simulink model "auto_pilot_udp"  (R2022b)
settings: Solver=FixedStepAuto  StartTime=0.0  StopTime=Inf  FixedStep=0.001  RelTol=1e-3  EnableMultiTasking=on
InitFcn:
  | clear mex
model workspace (MAT data in the model file):
  worldsim_instance : object (value not decoded)
values from neighbouring files (symbols this model uses):
  ACC_Adaptive_D = 0    [AutoPilot_parameters.m]    (also in ap_ini_param.mat; ap_initialModel.sldd = 0.0)
  ACC_Adaptive_I = 0    [AutoPilot_parameters.m]    (also in ap_ini_param.mat; ap_initialModel.sldd = 0.0)
  ACC_Adaptive_P = [5 7.5]    [AutoPilot_parameters.m]    (also in ap_ini_param.mat; ap_initialModel.sldd = 5.0 7.5)
  ACC_Classic_I = 5    [AutoPilot_parameters.m]    (also in ap_ini_param.mat; ap_initialModel.sldd = 5.0)
  ACC_Classic_P = 15    [AutoPilot_parameters.m]    (also in ap_ini_param.mat; ap_initialModel.sldd = 15.0)
  ACC_MaxBrake = 50    [AutoPilot_parameters.m]    (also in ap_ini_param.mat; ap_initialModel.sldd = 50.0)
  ACC_MaxThrottle = 130    [AutoPilot_parameters.m]    (also in ap_ini_param.mat = 80; ap_initialModel.sldd = 130.0)
  ACC_Module_Activity_Flag = 1    [AutoPilot_parameters.m]    (also in ap_ini_param.mat; ap_initialModel.sldd = 1.0)
  ACC_Ready_Speed = 30    [AutoPilot_parameters.m]    (also in ap_ini_param.mat; ap_initialModel.sldd = 30.0)
  ACC_SensorMaxDistance = 250    [AutoPilot_parameters.m]    (also in ap_ini_param.mat = 120; ap_initialModel.sldd = 250.0)
  ACC_Speed_Distance_control = 3    [AutoPilot_parameters.m]    (also in ap_ini_param.mat; ap_initialModel.sldd = 3.0)
  ACC_Speed_Distance_Gain = [0.1 0.15 0.2 0.25]    [AutoPilot_parameters.m]    (also in ap_ini_param.mat; ap_initialModel.sldd = 0.1 0.15 0.2 0.25)
  ADAS_Control_Mode = 1    [AutoPilot_parameters.m]    (also in ap_ini_param.mat; ap_initialModel.sldd = 1.0)
  AEB_Alarm_Freq = 5    [AutoPilot_parameters.m]    (also in ap_ini_param.mat; ap_initialModel.sldd = 5.0)
  AEB_Distance_To_Collision_Brake = 5    [AutoPilot_parameters.m]    (also in ap_ini_param.mat; ap_initialModel.sldd = 5.0)
  AEB_Freq_Hz = Sensor_Freq_worldsim/2    (= 25)    [AutoPilot_parameters.m]    (also in ap_ini_param.mat; ap_initialModel.sldd = 25.0)
  AEB_Gain = [1 1]    [AutoPilot_parameters.m]    (also in ap_ini_param.mat; ap_initialModel.sldd = 1.0 1.0)
  AEB_Gain_set = 60    [AutoPilot_parameters.m]    (also in ap_ini_param.mat; ap_initialModel.sldd = 60.0)
  AEB_Gain_set_mult = 0.03    [AutoPilot_parameters.m]    (also in ap_ini_param.mat; ap_initialModel.sldd)
  AEB_Max_Decel = [8 15]    [AutoPilot_parameters.m]    (also in ap_ini_param.mat; ap_initialModel.sldd = 8.0 15.0)
  AEB_Max_Speed = 150    [AutoPilot_parameters.m]    (also in ap_ini_param.mat = 100; ap_initialModel.sldd = 150.0)
  AEB_Min_Distance_at_Stop = 1    [AutoPilot_parameters.m]    (also in ap_ini_param.mat; ap_initialModel.sldd = 1.0)
  AEB_Module_Activity_Flag = 1    [AutoPilot_parameters.m]    (also in ap_ini_param.mat; ap_initialModel.sldd = 1.0)
  AEB_Pedestrian_type = 68    [AutoPilot_parameters.m]    (also in ap_ini_param.mat; ap_initialModel.sldd = 68.0)
  AEB_Steer_Max = 180    [AutoPilot_parameters.m]    (also in ap_ini_param.mat; ap_initialModel.sldd = 180.0)
  AP_Activity_Flag = 1    [AutoPilot_parameters.m]    (also in ap_ini_param.mat; ap_initialModel.sldd = 1.0)
  AP_D = [0.3 0.3]    [AutoPilot_parameters.m]    (also in ap_ini_param.mat; ap_initialModel.sldd = 0.3 0.3)
  AP_Dyn_Rate_Limiter_Gain = 0.1    [AutoPilot_parameters.m]    (also in ap_ini_param.mat; ap_initialModel.sldd)
  AP_Dyn_Rate_Limiter_Power = 10    [AutoPilot_parameters.m]    (also in ap_ini_param.mat; ap_initialModel.sldd = 10.0)
  AP_Error_Max = 3    [AutoPilot_parameters.m]    (also in ap_ini_param.mat; ap_initialModel.sldd = 3.0)
  AP_Freq_Hz = Sensor_Freq_worldsim    (= 50)    [AutoPilot_parameters.m]    (also in ap_ini_param.mat; ap_initialModel.sldd = 50.0)
  AP_I = [0.05 0.05]    [AutoPilot_parameters.m]    (also in ap_ini_param.mat; ap_initialModel.sldd = 0.05 0.05)
  AP_Max_Error_dydt_Disable = 0.5    [AutoPilot_parameters.m]    (also in ap_ini_param.mat; ap_initialModel.sldd)
  AP_On_Request_Time = 0.01    [AutoPilot_parameters.m]    (also in ap_ini_param.mat; ap_initialModel.sldd)
  AP_P = [0.2 0.2]    [AutoPilot_parameters.m]    (also in ap_ini_param.mat; ap_initialModel.sldd = 0.2 0.2)
  AP_Steer_Error_Max = 0.7    [AutoPilot_parameters.m]    (also in ap_ini_param.mat; ap_initialModel.sldd)
  AP_Steer_Rate_Max_radps = 1    [AutoPilot_parameters.m]    (also in ap_ini_param.mat; ap_initialModel.sldd = 1.0)
  AP_Transition_Rate = 0.5    [AutoPilot_parameters.m]    (also in ap_ini_param.mat; ap_initialModel.sldd)
  butter_a = [1 -1.9911142922 0.991153595869]    [ap_ini_param.mat]    (also in ap_initialModel.sldd = 1.0 -1.9911142922016536 0.99115359586893548)
  butter_a_lka_out = 1.0 -1.5610180758007179 0.641351538057563    [ap_initialModel.sldd]
  butter_b = [9.82591682048e-06 1.9651833641e-05 9.82591682048e-06]    [ap_ini_param.mat]    (also in ap_initialModel.sldd = 9.825916820482009E-6 1.9651833640964018E-5 9.825916820482009)
  butter_b_lka_out = 0.020083365564211246 0.040166731128422492 0.020083365564211246    [ap_initialModel.sldd]
  Lane_Width = 3.7    [AutoPilot_parameters.m]    (also in ap_ini_param.mat; ap_initialModel.sldd)
  LDW_Activity_Flag = 1    [ap_ini_param.mat]    (also in ap_initialModel.sldd = 1.0)
  LDW_Freq_Hz = 50    [ap_ini_param.mat]    (also in ap_initialModel.sldd = 50.0)
  LDW_LaneGap_dydt_Warning = 50    [ap_ini_param.mat]    (also in ap_initialModel.sldd = 50.0)
  LDW_LaneGap_Warning = [0.5 0.25]    [ap_ini_param.mat]    (also in ap_initialModel.sldd = 0.5 0.25)
  LDW_Min_Speed = 60    [ap_ini_param.mat]    (also in ap_initialModel.sldd = 60.0)
  LDW_Steer_Vibration_Amplitude = 5    [ap_ini_param.mat]    (also in ap_initialModel.sldd = 5.0)
  LDW_Steer_Vibration_Freq = 25    [ap_ini_param.mat]    (also in ap_initialModel.sldd = 25.0)
  LKA_Activity_Flag = 1    [ap_ini_param.mat]    (also in ap_initialModel.sldd = 1.0)
  LKA_D = [0.2 0.3]    [ap_ini_param.mat]    (also in ap_initialModel.sldd = 0.2 0.3)
  LKA_Dyn_Rate_Limiter_Gain = 0.1    [ap_ini_param.mat]    (also in ap_initialModel.sldd)
  LKA_Dyn_Rate_Limiter_Power = 10    [ap_ini_param.mat]    (also in ap_initialModel.sldd = 10.0)
  LKA_Error_dydt_Off = 1    [ap_ini_param.mat]    (also in ap_initialModel.sldd = 1.0)
  LKA_Error_Max = 3    [ap_ini_param.mat]    (also in ap_initialModel.sldd = 3.0)
  LKA_Error_Off = 0.5    [ap_ini_param.mat]    (also in ap_initialModel.sldd)
  LKA_Freq_Hz = 50    [ap_ini_param.mat]    (also in ap_initialModel.sldd = 50.0)
  LKA_I = [0.025 0.05]    [ap_ini_param.mat]    (also in ap_initialModel.sldd = 0.025 0.05)
  LKA_Lane_Gap_Activate = [0.25 0.125]    [ap_ini_param.mat]    (also in ap_initialModel.sldd = 0.25 0.125)
  LKA_Lane_Gap_dydt_Activate = 50    [ap_ini_param.mat]    (also in ap_initialModel.sldd = 50.0)
  LKA_Min_Speed = 60    [ap_ini_param.mat]    (also in ap_initialModel.sldd = 60.0)
  LKA_On_Display_Freq = 5    [ap_ini_param.mat]    (also in ap_initialModel.sldd = 5.0)
  LKA_P = [0.1 0.2]    [ap_ini_param.mat]    (also in ap_initialModel.sldd = 0.1 0.2)
  LKA_Steer_Rate_Max_radps = 1    [ap_ini_param.mat]    (also in ap_initialModel.sldd = 1.0)
  No_Target_Display_Value = 0    [AutoPilot_parameters.m]    (also in ap_ini_param.mat; ap_initialModel.sldd = 0.0)
  radar_source = 2    [AutoPilot_parameters.m]    (also in ap_ini_param.mat; ap_initialModel.sldd = 2.0)
  Sensor_Freq_worldsim = 50    [AutoPilot_parameters.m]    (also in ap_ini_param.mat; ap_initialModel.sldd = 50.0; launcher.m)
  stop_number_collisions = 10.0    [ap_initialModel.sldd]    (also in launcher.m = 10)
  stop_speed = 0.001    [ap_initialModel.sldd]    (also in launcher.m)
  stop_time = 12.0    [ap_initialModel.sldd]    (also in launcher.m = 12)
  vehicle_width = 2.2    [AutoPilot_parameters.m]    (also in ap_ini_param.mat = 1.86; ap_initialModel.sldd)
undefined symbols (not defined in the file or in its folder): blockPlatform, HOST, light_brake_center, light_brake_left, light_brake_right
libraries: simulink x103, simwbSfunlib x35, slpidlib x5, viworldsim_lib x5
(part 2 of 5)

== system auto_pilot_udp/To_SimWB_Host1 ==
  VI_CarRealTime.Inputs.Driver_Demands.str_swa : Inport
  VI_CarRealTime.Inputs.steer_assist.torque : Inport  Port=2
  VI_CarRealTime.Inputs.Driver_Demands.throttle : Inport  Port=3
  VI_CarRealTime.Inputs.Driver_Demands.brake : Inport  Port=4
  Byte Pack : S-Function  FunctionName=any2byte  Parameters=datatypesout,byteAlign  SFunctionDeploymentMode=off  EnableBusSupport=off  mask(Byte pack){datatypes={'double','double','double','double'}, byteAlign=1}
      mask prompts: datatypes "Input port data types (cell array):"; byteAlign "Byte alignment:"
      mask help: Pack input data into a single output vector of type uint8. Insert before a UDP Send block to produce a uint8 byte vector from multiple vectors of varying data type.
      mask init:
      | datatypesout = bytepack_callback(datatypes);
      mask Help: eval('linkfoundation.util.blockHelpLink(''ecoder'')');
      mask TypeOptions byteAlign: 1 | 2 | 4 | 8
      mask Display:
      | color('blue');
      | text(0.95, 0.90, '', ...
      |                 'horizontalalignment', 'right');
      | color('black');
      | text(0.50, 0.12, 'Byte Pack', ...
      |                 'horizontalAlignment','center');
  UDP Send : S-Function  FunctionName=sdspToNetwork  Parameters=localURL, localPortSource, localPort, remoteURL, remotePort, sendBufferSize, separateLengthPort, []  SFunctionDeploymentMode=off  EnableBusSupport=off  mask(UDP Send){remoteURL=remoteURL, remotePort=remotePort, localURL='255.255.255.255', localPortSource=Automatically determine, localPort=-1, sendBufferSize=8192, sampletime=-1, blockPlatform=blockPlatform, separateLengthPort=0}
      mask prompts: remoteURL "Remote IP address ('255.255.255.255' for broadcast):"; remotePort "Remote IP port:"; localURL "Local IP address:"; localPortSource "Local IP port source:"; localPort "Local IP port:"; sendBufferSize "Send buffer size (bytes):"; blockPlatform "Block Platform"; separateLengthPort "Use a separate length port"
      mask help: Send a UDP packet to a network address identified by the remote IP address and remote IP port parameters.
      mask Help: eval('dspnetwork_help(''UDPSend'')')
      mask TypeOptions localPortSource: Automatically determine | Specify via dialog
      mask Callback localPortSource:
      | mask_vis = get_param(gcbh, 'MaskVisibilities');
      | if strcmp(get_param(gcbh,'localPortSource'),'Specify via dialog')
      |     mask_vis{5} = 'on';
      | else
      |     mask_vis{5} = 'off';
      | end
      | set_param(gcbh, 'MaskVisibilities', mask_vis);
      | clear('mask_vis');
      mask Display:
      | fprintf('UDP Send');
      | color('blue');
      | text(0.97, 0.87, get_param(gcb, 'blockPlatform'), 'horizontalalignment', 'right');
  wires:
  Byte Pack/1 -> UDP Send/1
  VI_CarRealTime.Inputs.Driver_Demands.str_swa/1 -> Byte Pack/1
  VI_CarRealTime.Inputs.steer_assist.torque/1 -> Byte Pack/2
  VI_CarRealTime.Inputs.Driver_Demands.throttle/1 -> Byte Pack/3
  VI_CarRealTime.Inputs.Driver_Demands.brake/1 -> Byte Pack/4

== system auto_pilot_udp/VI-WorldSim Lights Manager ==
  light_brake_left : Inport
  light_brake_right : Inport  Port=2
  light_brake_center : Inport  Port=3
  Lights : Subsystem
  Lights Bus : Outport  VectorParamsAs1DForOutWhenUnconnected=off
  wires:
  Lights/1(Out1) -> Lights Bus/1
  light_brake_left/1 -> Lights/1(light_brake_left)
  light_brake_right/1 -> Lights/2(light_brake_right)
  light_brake_center/1 -> Lights/3(light_brake_center)

== system auto_pilot_udp/ACC/ACC_Inputs ==
  note: additional speed increase
  ADAS_map : Subsystem
  Cast To Double : DataTypeConversion  OutDataTypeStr=double  SaturateOnIntegerOverflow=off  RndMeth=Floor
  Clock : Clock
  Compare To Constant : simulink/Logic and Bit Operations/Compare To Constant  relop=>=  const=1.5  OutDataTypeStr=boolean
  Constant : Constant  Value=300
  Constant1 : Constant  Value=0
  Constant2 : Constant
  Constant3 : Constant
  Detect Increase : simulink/Logic and Bit Operations/Detect Increase  vinit=0.0  OutDataTypeStr=boolean
  Divide : Product  Inputs=*/
  Gain1 : Gain  Gain=-1
  Logical Operator : Logic  Operator=OR  AllPortsSameDT=off  OutDataTypeStr=boolean
  Sum : Sum
  tag scope: ACC_Input_ACC_On_Request=global, ACC_Input_AEB_Output_Active=global, ACC_Input_Driver_Brake=global, ACC_Input_Driver_Throttle=global, ACC_Input_Front_Axle_Steer=global, ACC_Input_Vehicle_Speed=global, ACC_Input_Vicrt_Status=global, Additional_speed=global, Vicrt_Status=global, reset_ACC=global
  wires:
  [Driver_Brake] -> [ACC_Input_Driver_Brake]
  [Driver_Throttle] -> [ACC_Input_Driver_Throttle]
  [AEB_Output_Active] -> [ACC_Input_AEB_Output_Active]
  [Vehicle_Speed] -> [ACC_Input_Vehicle_Speed]
  Constant2/1 -> [Vicrt_Status], [ACC_Input_Vicrt_Status]
  [Front_Axle_Steer] -> [ACC_Input_Front_Axle_Steer]
  Logical Operator/1 -> [ACC_Input_ACC_On_Request]
  [plus] -> Sum/1
  [minus] -> Gain1/1
  Sum/1 -> Divide/1
  Gain1/1 -> Sum/2
  [set_acc_plus] -> Logical Operator/1
  [AP_Input_LK_On_Request] -> Logical Operator/2
  Divide/1 -> [Additional_speed]
  Constant/1 -> Divide/2
  [res] -> [reset_ACC]
  Constant1/1 -> ADAS_map/4(ACC_engage/ACC_speed_increase), ADAS_map/6(ACC_cancel), ADAS_map/5(ACC_speed_decrease), ADAS_map/3(ACC_reset), ADAS_map/2(ACC_distance_increase), ADAS_map/1(ACC_distance_decrease)
  Clock/1 -> Compare To Constant/1
  Compare To Constant/1 -> Detect Increase/1
  Detect Increase/1 -> Cast To Double/1
  Cast To Double/1 -> ADAS_map/7(AutoPilot_engage)
  Constant3/1 -> [AEB_Output_Active]

== system auto_pilot_udp/ACC/ACC_Logic ==
  ACC_Speed_Controller : Subsystem
  ACC_Switch : Subsystem
  ACC_Target_Acquisition : Subsystem

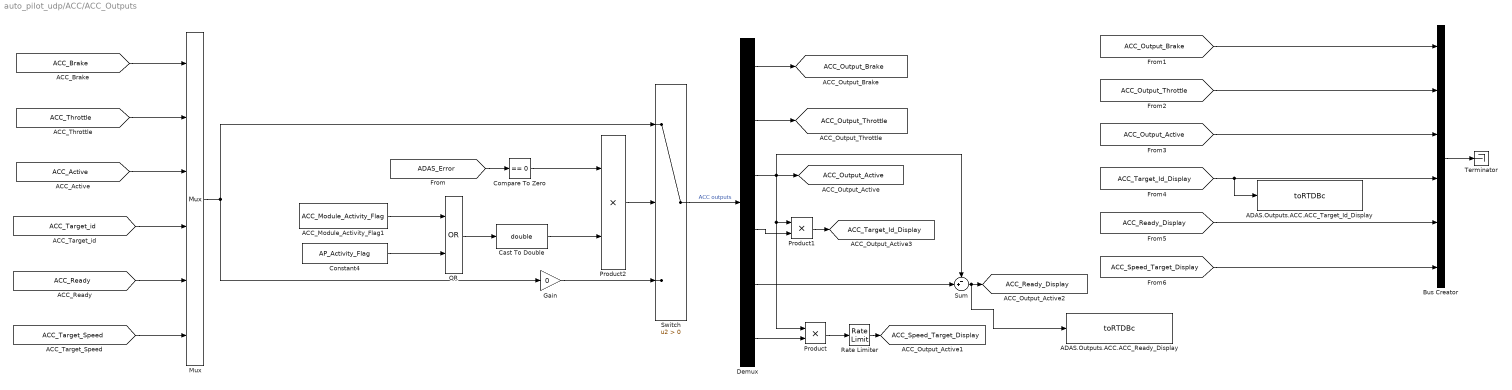
== system auto_pilot_udp/ACC/ACC_Outputs ==
  ACC_Module_Activity_Flag1 : Constant  Value=ACC_Module_Activity_Flag
  ADAS.Outputs.ACC.ACC_Ready_Display : simwbSfunlib/toRTDBc  stringBlock=off  varName=ADAS.Outputs.ACC.ACC_Ready_Display  sigDim=[1 1]  sigType=double  sampleTime=[-1 0]  maxBuffSize=1024  busName=nobus  defaultValue=0  defaultString=simwbout  hasMapping=0  ptrName=ADAS_Outputs_ACC_ACC_Ready_Display  enumOrAlias=nothing
      settings: SourceProductName=SimWB MLToolkit
  ADAS.Outputs.ACC.ACC_Target_Id_Display : simwbSfunlib/toRTDBc  stringBlock=off  varName=ADAS.Outputs.ACC.ACC_Target_Id_Display  sigDim=[1 1]  sigType=double  sampleTime=[-1 0]  maxBuffSize=1024  busName=nobus  defaultValue=0  defaultString=simwbout  hasMapping=0  ptrName=ADAS_Outputs_ACC_ACC_Target_Id_Display  enumOrAlias=nothing
      settings: SourceProductName=SimWB MLToolkit
  Bus Creator : BusCreator  Inputs=6
  Cast To Double : DataTypeConversion  OutDataTypeStr=double  SaturateOnIntegerOverflow=off  RndMeth=Floor
  Compare To Zero : simulink/Logic and Bit Operations/Compare To Zero  relop===  OutDataTypeStr=boolean
  Constant4 : Constant  Value=AP_Activity_Flag
  Demux : Demux  Outputs=6
  Gain : Gain  Gain=0
  Mux : Mux  Inputs=6
  OR : Logic  Operator=OR  AllPortsSameDT=off  OutDataTypeStr=boolean
  Product : Product
  Product1 : Product
  Product2 : Product
  Rate Limiter : RateLimiter  RisingSlewLimit=inf  FallingSlewLimit=-100  SampleTimeMode=inherited
  Sum : Sum  Inputs=-+|
  Switch : Switch  Criteria=u2 > Threshold  SaturateOnIntegerOverflow=off  InputSameDT=off
  Terminator : Terminator
  tag scope: ACC_Output_Active=global, ACC_Output_Brake=global, ACC_Output_Throttle=global, ACC_Ready_Display=global, ACC_Speed_Target_Display=global, ACC_Target_Id_Display=global
  wires:
  [ACC_Brake] -> Mux/1
  [ACC_Throttle] -> Mux/2
  Mux/1 -> Switch/1, Gain/1
  Switch/1 -> Demux/1  "ACC outputs"
  Cast To Double/1 -> Product2/2
  Demux/1 -> [ACC_Output_Brake]
  Demux/2 -> [ACC_Output_Throttle]
  Gain/1 -> Switch/3
  [ACC_Active] -> Mux/3
  [ACC_Target_id] -> Mux/4
  Demux/4 -> Product1/2
  [ACC_Ready] -> Mux/5
  [ACC_Target_Speed] -> Mux/6
  Demux/5 -> Sum/2
  Demux/6 -> Product/2
  Product/1 -> Rate Limiter/1
  [ADAS_Error] -> Compare To Zero/1
  Product2/1 -> Switch/2
  Compare To Zero/1 -> Product2/1
  ACC_Module_Activity_Flag1/1 -> OR/1
  Constant4/1 -> OR/2
  OR/1 -> Cast To Double/1
  Demux/3 -> Sum/1, Product/1, Product1/1, [ACC_Output_Active]
  Rate Limiter/1 -> [ACC_Speed_Target_Display]
  Sum/1 -> ADAS.Outputs.ACC.ACC_Ready_Display/1, [ACC_Ready_Display]
  Product1/1 -> [ACC_Target_Id_Display]
  [ACC_Output_Brake] -> Bus Creator/1
  [ACC_Output_Throttle] -> Bus Creator/2
  [ACC_Output_Active] -> Bus Creator/3
  [ACC_Target_Id_Display] -> Bus Creator/4, ADAS.Outputs.ACC.ACC_Target_Id_Display/1
  [ACC_Ready_Display] -> Bus Creator/5
  [ACC_Speed_Target_Display] -> Bus Creator/6
  Bus Creator/1 -> Terminator/1

== system auto_pilot_udp/AEB/AEB_Inputs ==
  Gain{,1..3} (4 alike) : Gain  Gain=0
  Gain4 : Gain  Gain=-1
  Gain5 : Gain  Gain=-1
  MATLAB Function : MATLAB Function  TreatAsAtomicUnit=on
  MATLAB Function1 : MATLAB Function  TreatAsAtomicUnit=on
  Mux{,1..3} (4 alike) : Mux  Inputs=3
  tag scope: AEB_Input_Driver_Steering=global, AEB_Input_SensorTargets_azimuthInSensor_mux=global, AEB_Input_SensorTargets_distanceToCollision_mux=global, AEB_Input_SensorTargets_id_mux=global, AEB_Input_SensorTargets_type_mux=global, AEB_Input_Vehicle_Speed=global
  wires:
  [SensorTargets_300002_distanceToCollision_mux] -> MATLAB Function1/1(u)
  [SensorTargets_300001_distanceToCollision_mux] -> MATLAB Function/1(u)
  [SensorTargets_300000_distanceToCollision_mux] -> Gain/1
  [SensorTargets_300001_id_mux] -> Mux1/2
  [SensorTargets_300000_id_mux] -> Gain1/1
  [SensorTargets_300000_azimuthInSensor_mux] -> Gain2/1
  [SensorTargets_300001_azimuthInSensor_mux] -> Gain4/1
  [SensorTargets_300002_azimuthInSensor_mux] -> Gain5/1
  MATLAB Function1/1(y) -> Mux/3
  [SensorTargets_300002_id_mux] -> Mux1/3
  Gain5/1 -> Mux2/3
  [Driver_Steering] -> [AEB_Input_Driver_Steering]
  [Vehicle_Speed] -> [AEB_Input_Vehicle_Speed]
  [SensorTargets_300001_type_mux] -> Mux3/2
  [SensorTargets_300000_type_mux] -> Gain3/1
  [SensorTargets_300002_type_mux] -> Mux3/3
  Gain/1 -> Mux/1
  Gain1/1 -> Mux1/1
  Gain2/1 -> Mux2/1
  Gain3/1 -> Mux3/1
  MATLAB Function/1(y) -> Mux/2
  Gain4/1 -> Mux2/2
  Mux/1 -> [AEB_Input_SensorTargets_distanceToCollision_mux]
  Mux1/1 -> [AEB_Input_SensorTargets_id_mux]
  Mux2/1 -> [AEB_Input_SensorTargets_azimuthInSensor_mux]
  Mux3/1 -> [AEB_Input_SensorTargets_type_mux]

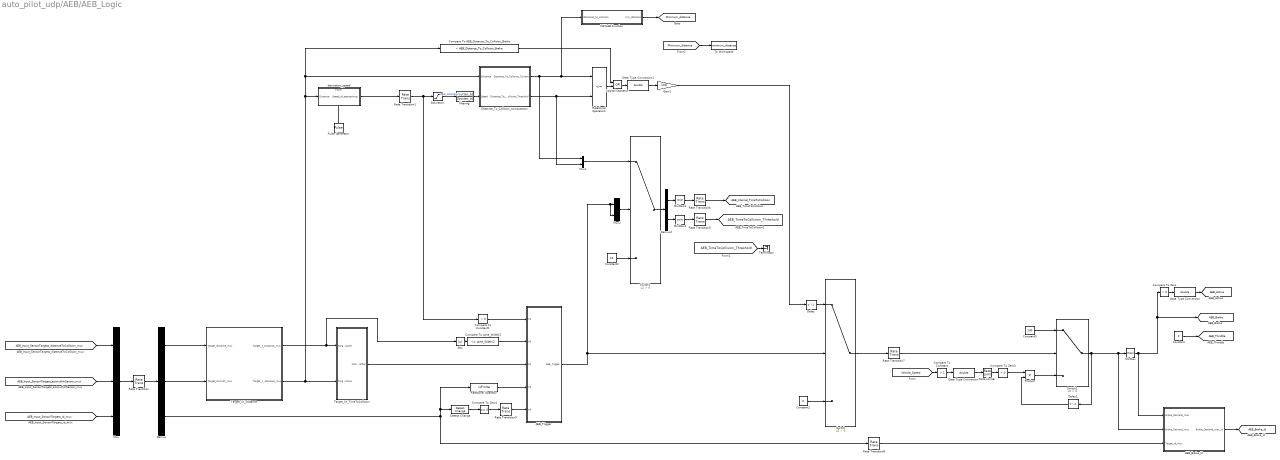
== system auto_pilot_udp/AEB/AEB_Logic ==
  "AEB_Brake_id " : Subsystem
  AEB_Trigger : Subsystem
  Abs : Abs  SaturateOnIntegerOverflow=off
  Compare To AEB_Distance_To_Collision_Brake : simulink/Logic and Bit Operations/Compare To Constant  relop=<  const=AEB_Distance_To_Collision_Brake  OutDataTypeStr=boolean
  Compare To Constant : simulink/Logic and Bit Operations/Compare To Constant  relop=>  const=1  OutDataTypeStr=boolean
  Compare To Constant1 : simulink/Logic and Bit Operations/Compare To Constant  relop=>  const=0  OutDataTypeStr=boolean
  Compare To Lane_Width/2 : simulink/Logic and Bit Operations/Compare To Constant  relop=<=  const=Lane_Width/2  OutDataTypeStr=boolean
  Compare To Zero : simulink/Logic and Bit Operations/Compare To Zero  relop=>  OutDataTypeStr=boolean
  Compare To Zero1 : simulink/Logic and Bit Operations/Compare To Zero  relop===  OutDataTypeStr=boolean
  Compare To Zero3 : simulink/Logic and Bit Operations/Compare To Zero  relop=>  OutDataTypeStr=boolean
  Constant : Constant  Value=0
  Constant1 : Constant  Value=0
  Constant2 : Constant  Value=10
  Constant3 : Constant  Value=100
  Data Type Conversion : DataTypeConversion  OutDataTypeStr=double  SaturateOnIntegerOverflow=off  RndMeth=Floor
  Data Type Conversion1 : DataTypeConversion  OutDataTypeStr=double  SaturateOnIntegerOverflow=off  RndMeth=Floor
  Data Type Conversion2 : DataTypeConversion  OutDataTypeStr=double  SaturateOnIntegerOverflow=off  RndMeth=Floor
  Delay : Delay  DelayLength=1  InitialCondition=0
  Delay1 : Delay  DelayLength=1
  Demux : Demux  Outputs=3
  Demux2 : Demux  Outputs=2
  Detect Change : simulink/Logic and Bit Operations/Detect Change  vinit=0  OutDataTypeStr=boolean
  Distance_To_Collision_computation : Subsystem
  Gain1 : Gain  Gain=100
  Logical Operator : Logic  Operator=OR  AllPortsSameDT=off  OutDataTypeStr=boolean
  MATLAB Function : MATLAB Function  TreatAsAtomicUnit=on
  MinMax : MinMax  Function=max
  MinMax3 : MinMax
  MinMax4 : MinMax
  Mux : Mux  Inputs=3
  Mux1 : Mux  Inputs=2
  Mux2 : Mux  Inputs=2
  Product : Product
  Pulse Generator : DiscretePulseGenerator  PulseType=Time based  Period=1/AEB_Freq_Hz  PulseWidth=2.5
  Rate Limiter : RateLimiter  RisingSlewLimit=inf  SampleTimeMode=inherited
  Rate Transition{,1,8..9} (4 alike) : RateTransition  OutPortSampleTime=1/AEB_Freq_Hz
  Rate Transition5 : RateTransition  OutPortSampleTime=1/1000
  Rate Transition6 : RateTransition  OutPortSampleTime=1/1000
  Rate Transition7 : RateTransition  OutPortSampleTime=1/1000
  Relational Operator : RelationalOperator  Operator=isFinite  OutDataTypeStr=boolean  InputSameDT=off
  Relational Operator1 : RelationalOperator  Operator=<=  OutDataTypeStr=boolean  InputSameDT=off
  Saturation : Saturate  UpperLimit=inf  LowerLimit=1e-6
  Switch : Switch  Criteria=u2 > Threshold  SaturateOnIntegerOverflow=off  InputSameDT=off
  Switch1 : Switch  Criteria=u2 > Threshold  SaturateOnIntegerOverflow=off  InputSameDT=off
  Switch2 : Switch  Criteria=u2 > Threshold  SaturateOnIntegerOverflow=off  InputSameDT=off
  Target_XY_Distance : MATLAB Function  TreatAsAtomicUnit=on
  Target_XY_TimeToCollision : Subsystem
  Terminator : Terminator
  To Workspace : ToWorkspace  VariableName=minimum_distance  SampleTime=-1
      settings: Save2DSignal=2-D array (concatenate along first dimension)
  derivation_speed : Subsystem
  filtering : DiscreteFilter  Numerator=[butter_b]  Denominator=[butter_a]  SampleTime=1e-3
  tag scope: AEB_Active=global, AEB_Brake=global, AEB_Brake_id=global, AEB_Internal_TimeToCollision=global, AEB_Throttle=global, AEB_TimeToCollision_Threshold=global, Minimum_distance=global
  wires:
  [AEB_Input_SensorTargets_distanceToCollision_mux] -> Mux/1
  [AEB_Input_SensorTargets_azimuthInSensor_mux] -> Mux/2
  Mux/1 -> Rate Transition/1
  Compare To Zero/1 -> Data Type Conversion/1
  [AEB_Input_SensorTargets_id_mux] -> Mux/3
  Constant1/1 -> Switch/3
  Rate Transition/1 -> Demux/1
  Switch/1 -> Rate Transition7/1
  Distance_To_Collision_computation/2(Distance_To_Collision_Threshold) -> Mux1/2, Relational Operator1/2
  Distance_To_Collision_computation/1(Distance_To_Collision_Current) -> Mux1/1, MATLAB Function/1(distances_to_collision), Relational Operator1/1
  Gain1/1 -> Delay/1
  Constant2/1 -> Switch1/3
  MinMax3/1 -> Rate Transition6/1
  Data Type Conversion1/1 -> Gain1/1
  Saturation/1 -> filtering/1  "after_saturation"
  MinMax4/1 -> Rate Transition5/1
  Mux1/1 -> Switch1/1
  Mux2/1 -> Switch1/2
  Switch1/1 -> Demux2/1
  Demux2/1 -> MinMax3/1
  Demux2/2 -> MinMax4/1
  Detect Change/1 -> Compare To Zero1/1
  "AEB_Brake_id "/1(Brake_Demand_max_id) -> [AEB_Brake_id]
  MinMax/1 -> "AEB_Brake_id "/1(Brake_Demand_max), [AEB_Brake], Compare To Zero/1
  Data Type Conversion/1 -> [AEB_Active]
  Constant/1 -> [AEB_Throttle]
  Rate Transition5/1 -> [AEB_TimeToCollision_Threshold]
  Rate Transition6/1 -> [AEB_Internal_TimeToCollision]
  Target_XY_TimeToCollision/1(Collision_Identifier) -> AEB_Trigger/3(In2)
  Compare To Zero1/1 -> Rate Transition9/1
  Target_XY_Distance/1(Target_Y_Distance_mux) -> Abs/1, Target_XY_TimeToCollision/1(Target_Y_Distance)
  Abs/1 -> Compare To Lane_Width/2/1
  Relational Operator1/1 -> Logical Operator/2
  Compare To AEB_Distance_To_Collision_Brake/1 -> Logical Operator/1
  Delay/1 -> Switch/1
  Switch2/1 -> Delay1/1, "AEB_Brake_id "/2(Brake_Demand_mux), MinMax/1
  Rate Transition8/1 -> "AEB_Brake_id "/3(Target_id_mux)
  Product/1 -> Switch2/3
  Delay1/1 -> Product/2
  [Vehicle_Speed] -> Compare To Constant/1
  Compare To Constant/1 -> Data Type Conversion2/1
  Rate Transition7/1 -> Switch2/2
  Constant3/1 -> Switch2/1
  Compare To Zero3/1 -> Product/1
  Rate Limiter/1 -> Compare To Zero3/1
  Data Type Conversion2/1 -> Rate Limiter/1
  AEB_Trigger/1(AEB_Trigger) -> Switch/2, Mux2/1, Mux2/2
  Demux/3 -> Relational Operator/1, Detect Change/1, Rate Transition8/1
  Demux/1 -> Target_XY_Distance/1(Target_distance_mux)
  Demux/2 -> Target_XY_Distance/2(Target_azimuth_mux)
  Compare To Constant1/1 -> AEB_Trigger/1(In1)
  Rate Transition9/1 -> AEB_Trigger/5(In4)
  Compare To Lane_Width/2/1 -> AEB_Trigger/2(In5)
  Relational Operator/1 -> AEB_Trigger/4(In3)
  Logical Operator/1 -> Data Type Conversion1/1
  Target_XY_Distance/2(Target_X_Distance_mux) -> Target_XY_TimeToCollision/2(Target_X_Distance), Distance_To_Collision_computation/1(Distance), Compare To AEB_Distance_To_Collision_Brake/1, derivation_speed/1(Distance)
  [AEB_TimeToCollision_Threshold] -> Terminator/1
  Pulse Generator/1 -> derivation_speed/Trigger
  Rate Transition1/1 -> Compare To Constant1/1, Saturation/1
  derivation_speed/1(Speed_of_approaching) -> Rate Transition1/1
  filtering/1 -> Distance_To_Collision_computation/2(Speed)
  MATLAB Function/1(min_distance) -> [Minimum_distance]
  [Minimum_distance] -> To Workspace/1

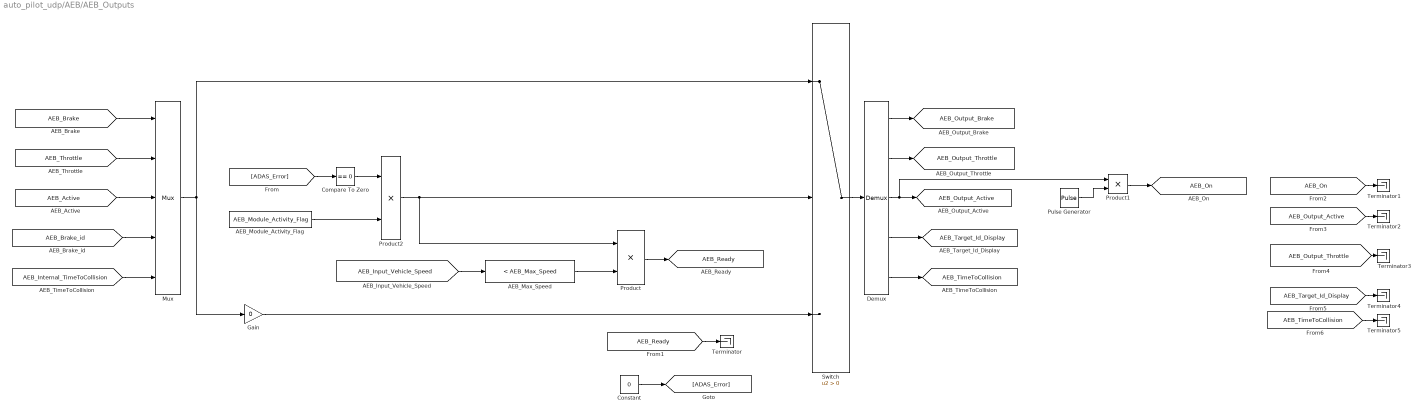
== system auto_pilot_udp/AEB/AEB_Outputs ==
  AEB_Max_Speed : simulink/Logic and Bit Operations/Compare To Constant  relop=<  const=AEB_Max_Speed  OutDataTypeStr=boolean
  AEB_Module_Activity_Flag : Constant  Value=AEB_Module_Activity_Flag
  Compare To Zero : simulink/Logic and Bit Operations/Compare To Zero  relop===  OutDataTypeStr=boolean
  Constant : Constant  Value=0
  Demux : Demux  Outputs=5
  Gain : Gain  Gain=0
  Mux : Mux  Inputs=5
  Product : Product
  Product1 : Product
  Product2 : Product
  Pulse Generator : DiscretePulseGenerator  PulseType=Time based  Period=1/AEB_Alarm_Freq  PulseWidth=50
  Switch : Switch  Criteria=u2 > Threshold  SaturateOnIntegerOverflow=off  InputSameDT=off
  Terminator{,1..5} (6 alike) : Terminator
  tag scope: AEB_On=global, AEB_Output_Active=global, AEB_Output_Brake=global, AEB_Output_Throttle=global, AEB_Ready=global, AEB_Target_Id_Display=global, AEB_TimeToCollision=global
  wires:
  [AEB_Brake] -> Mux/1
  [AEB_Throttle] -> Mux/2
  Mux/1 -> Switch/1, Gain/1
  Switch/1 -> Demux/1
  AEB_Module_Activity_Flag/1 -> Product2/2
  Demux/1 -> [AEB_Output_Brake]
  Demux/2 -> [AEB_Output_Throttle]
  Gain/1 -> Switch/3
  Demux/3 -> Product1/1, [AEB_Output_Active]
  [AEB_Active] -> Mux/3
  [AEB_Brake_id] -> Mux/4
  Demux/4 -> [AEB_Target_Id_Display]
  [AEB_Internal_TimeToCollision] -> Mux/5
  Demux/5 -> [AEB_TimeToCollision]
  [AEB_Input_Vehicle_Speed] -> AEB_Max_Speed/1
  AEB_Max_Speed/1 -> Product/2
  Pulse Generator/1 -> Product1/2
  [ADAS_Error] -> Compare To Zero/1
  Product2/1 -> Product/1, Switch/2
  Compare To Zero/1 -> Product2/1
  Product/1 -> [AEB_Ready]
  Product1/1 -> [AEB_On]
  [AEB_Ready] -> Terminator/1
  Constant/1 -> [ADAS_Error]
  [AEB_On] -> Terminator1/1
  [AEB_Output_Active] -> Terminator2/1
  [AEB_Output_Throttle] -> Terminator3/1
  [AEB_Target_Id_Display] -> Terminator4/1
  [AEB_TimeToCollision] -> Terminator5/1

== system auto_pilot_udp/AP/AP_Inputs ==
  Bus Creator : BusCreator  Inputs=2
  Demux : Demux  Outputs=2
  Gain4 : Gain  Gain=-1
  Mux4 : Mux  Inputs=2
  Terminator : Terminator
  tag scope: AP_Input_ACC_Ready=global, AP_Input_Driver_Brake=global, AP_Input_Driver_Steering=global, AP_Input_Driver_Throttle=global, AP_Input_LK_On_Request=global, AP_Input_laneGap_left=global, AP_Input_laneGap_right=global
  wires:
  [Driver_Steering] -> Gain4/1
  [mode] -> [AP_Input_LK_On_Request]
  [ACC_Ready] -> [AP_Input_ACC_Ready]
  [Driver_Brake] -> [AP_Input_Driver_Brake]
  [Driver_Throttle] -> [AP_Input_Driver_Throttle]
  [LaneGap_left_ws] -> Mux4/1
  Mux4/1 -> Demux/1
  [LaneGap_right_ws] -> Mux4/2
  Demux/1 -> [AP_Input_laneGap_left]
  Demux/2 -> [AP_Input_laneGap_right]
  Gain4/1 -> [AP_Input_Driver_Steering]
  [AP_Input_Driver_Brake] -> Bus Creator/1
  [AP_Input_Driver_Throttle] -> Bus Creator/2
  Bus Creator/1 -> Terminator/1

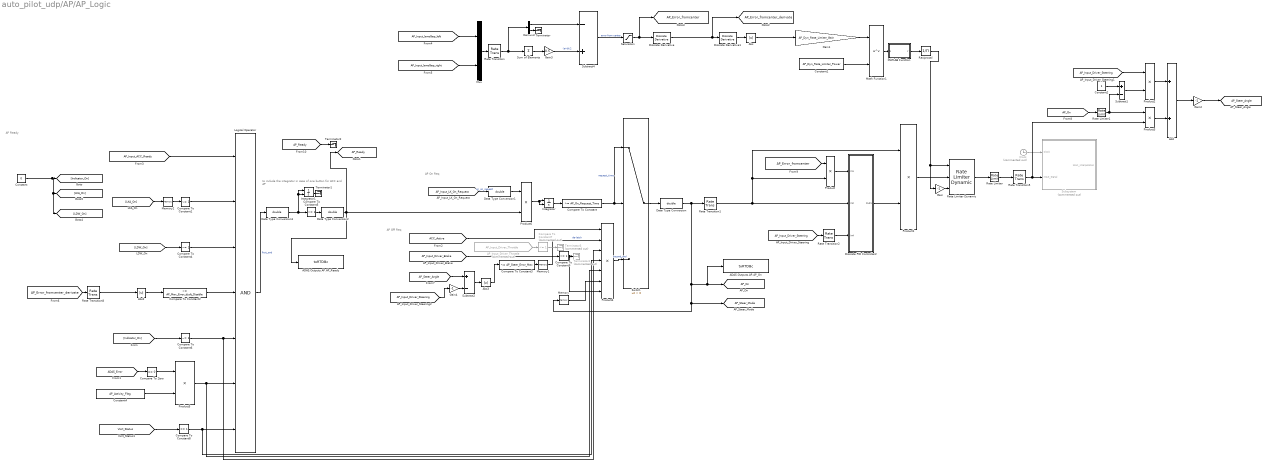
== system auto_pilot_udp/AP/AP_Logic ==
  note: to include the integrator in case of one button
      | for ACC and AP
  note: AP Off Req
  note: AP Ready
  note: AP On Req
  ADAS.Outputs.AP.AP_On : simwbSfunlib/toRTDBc  stringBlock=off  varName=ADAS.Outputs.AP.AP_On  sigDim=[1 1]  sigType=double  sampleTime=[-1 0]  maxBuffSize=1024  busName=nobus  defaultValue=0  defaultString=simwbout  hasMapping=0  ptrName=ADAS_Outputs_AP_AP_On  enumOrAlias=nothing
      settings: SourceProductName=SimWB MLToolkit
  ADAS.Outputs.AP.AP_Ready : simwbSfunlib/toRTDBc  stringBlock=off  varName=ADAS.Outputs.AP.AP_Ready  sigDim=[1 1]  sigType=double  sampleTime=[-1 0]  maxBuffSize=1024  busName=nobus  defaultValue=0  defaultString=simwbout  hasMapping=0  ptrName=ADAS_Outputs_AP_AP_Ready  enumOrAlias=nothing
      settings: SourceProductName=SimWB MLToolkit
  AP_Input_Driver_Throttle : From  Commented=on  GotoTag=AP_Input_Driver_Throttle  TagVisibility=global
  Abs : Abs  SaturateOnIntegerOverflow=off
  Abs2 : Abs  SaturateOnIntegerOverflow=off
  Abs3 : Abs  SaturateOnIntegerOverflow=off
  Add : Sum
  Clock : Clock  Commented=on
  Compare To Constant : simulink/Logic and Bit Operations/Compare To Constant  relop=>=  const=AP_On_Request_Time  OutDataTypeStr=boolean
  Compare To Constant1 : simulink/Logic and Bit Operations/Compare To Constant  relop=~=  const=1  OutDataTypeStr=boolean
  Compare To Constant2 : simulink/Logic and Bit Operations/Compare To Constant  relop=<=  const=AP_Max_Error_dydt_Disable  OutDataTypeStr=boolean
  Compare To Constant3 : simulink/Logic and Bit Operations/Compare To Constant  relop=<=  const=AP_Steer_Error_Max  OutDataTypeStr=boolean
  Compare To Constant4 : simulink/Logic and Bit Operations/Compare To Constant  relop=~=  const=1  OutDataTypeStr=boolean
  Compare To Constant5 : simulink/Logic and Bit Operations/Compare To Constant  relop=>=  const=1  OutDataTypeStr=boolean
  Compare To Constant6 : simulink/Logic and Bit Operations/Compare To Constant  relop=~=  const=1  OutDataTypeStr=boolean
  Compare To Constant7 : simulink/Logic and Bit Operations/Compare To Constant  Commented=on  relop=<=  const=1  OutDataTypeStr=boolean
  Compare To Constant8 : simulink/Logic and Bit Operations/Compare To Constant  relop===  const=1  OutDataTypeStr=boolean
  Compare To Constant9 : simulink/Logic and Bit Operations/Compare To Constant  relop=<=  const=1  OutDataTypeStr=boolean
  Compare To Zero : simulink/Logic and Bit Operations/Compare To Zero  relop===  OutDataTypeStr=boolean
  Constant : Constant  Value=0
  Constant1 : Constant  Value=AP_Dyn_Rate_Limiter_Power
  Constant2 : Constant
  Constant4 : Constant  Value=AP_Activity_Flag
  Data Type Conversion{,1..3} (4 alike) : DataTypeConversion  OutDataTypeStr=double  SaturateOnIntegerOverflow=off  RndMeth=Floor
  Demux3 : Demux  Outputs=2
  Discrete Derivative : simulink/Discrete/Discrete Derivative  gainval=1.0  ICPrevScaledInput=0.0  OutMin=[]  OutMax=[]  OutDataType=fixdt(1, 16)  OutScaling=2^-10  DoSatur=off
  Discrete Derivative1 : simulink/Discrete/Discrete Derivative  gainval=1.0  ICPrevScaledInput=0.0  OutMin=[]  OutMax=[]  OutDataType=fixdt(1, 16)  OutScaling=2^-10  DoSatur=off
  Discrete PID Controller2 : Subsystem
  Gain : Gain  Gain=-1
  Gain1 : Gain  Gain=AP_Dyn_Rate_Limiter_Gain
  Gain2 : Gain  Gain=-1
  Gain3 : Gain  Gain=0.5
  Gain4 : Gain  Gain=-1
  Integrator : Integrator  ExternalReset=either
  Integrator1 : Integrator  ExternalReset=either
  Logical Operator : Logic  Inputs=7  AllPortsSameDT=off  OutDataTypeStr=boolean
  MATLAB Function : MATLAB Function  TreatAsAtomicUnit=on
  Math Function1 : Math  Operator=pow  SignedPower=on
  Memory : Memory
  Memory1 : Memory
  Memory2 : Memory
  Mux : Mux  Inputs=2
  Product{,1..3,5..6} (6 alike) : Product
  Product4 : Product  Inputs=7
  Rate Limiter : RateLimiter  RisingSlewLimit=AP_Steer_Rate_Max_radps  FallingSlewLimit=-AP_Steer_Rate_Max_radps  SampleTimeMode=inherited
  Rate Limiter Dynamic : simulink/Discontinuities/Rate Limiter Dynamic
  Rate Limiter1 : RateLimiter  RisingSlewLimit=AP_Transition_Rate  FallingSlewLimit=-AP_Transition_Rate  SampleTimeMode=inherited
  Rate Transition : RateTransition  OutPortSampleTime=1/AP_Freq_Hz
  Rate Transition1 : RateTransition  OutPortSampleTime=1/AP_Freq_Hz
  Rate Transition2 : RateTransition  OutPortSampleTime=1/AP_Freq_Hz
  Rate Transition5 : RateTransition  OutPortSampleTime=1/1000
  Rate Transition8 : RateTransition  OutPortSampleTime=1/1000
  Reciprocal : Product  Inputs=/  RndMeth=Zero  SaturateOnIntegerOverflow=on
  Saturation : Saturate  UpperLimit=AP_Error_Max  LowerLimit=-AP_Error_Max
  Subsystem : Subsystem  Commented=on
  Subtract1 : Sum  Inputs=+-
  Subtract2 : Sum  Inputs=+-
  Subtract4 : Sum  Inputs=-+
  Sum of Elements : Sum  Inputs=+
  Switch : Switch  Criteria=u2 > Threshold  SaturateOnIntegerOverflow=off  InputSameDT=off
  Terminator : Terminator
  Terminator1 : Terminator
  Terminator2 : Terminator
  Terminator3 : Terminator  Commented=on
  Terminator4 : Terminator  Commented=on
  tag scope: AP_Error_fromcenter=global, AP_Error_fromcenter_derivate=global, AP_On=global, AP_Ready=global, AP_Steer_Angle=global, AP_Steer_Mode=global
  wires:
  Discrete Derivative/1 -> Discrete Derivative1/1, [AP_Error_fromcenter_derivate]
  Rate Transition1/1 -> Discrete PID Controller2/2(In2), Product1/1, Product/2
  Constant1/1 -> Math Function1/2
  Math Function1/1 -> MATLAB Function/1(u)
  Discrete Derivative1/1 -> Abs/1
  Gain1/1 -> Math Function1/1
  Reciprocal/1 -> Gain/1, Rate Limiter Dynamic/1
  Abs/1 -> Gain1/1
  Gain/1 -> Rate Limiter Dynamic/3
  Rate Limiter Dynamic/1 -> Rate Limiter/1
  Product1/1 -> Rate Limiter Dynamic/2
  Clock/1 -> Subsystem/1(Clock)
  Rate Limiter/1 -> Rate Transition5/1
  Saturation/1 -> [AP_Error_fromcenter], Discrete Derivative/1
  Constant2/1 -> Subtract1/1
  Subtract1/1 -> Product2/2
  Rate Limiter1/1 -> Subtract1/2, Product3/1
  Product2/1 -> Add/1
  Product3/1 -> Add/2
  Add/1 -> Gain2/1
  Subtract2/1 -> Abs3/1
  [AP_Input_LK_On_Request] -> Data Type Conversion1/1  "LK_on_request"
  Switch/1 -> Data Type Conversion/1
  Product4/1 -> Switch/3  "second_and"
  Data Type Conversion/1 -> Memory/1, [AP_Steer_Mode], ADAS.Outputs.AP.AP_On/1, [AP_On], Rate Transition1/1
  Data Type Conversion1/1 -> Product6/1
  Rate Transition8/1 -> Abs2/1
  Abs2/1 -> Compare To Constant2/1
  Compare To Constant2/1 -> Logical Operator/4
  Abs3/1 -> Compare To Constant3/1
  Compare To Constant3/1 -> Memory1/1
  [LDW_On] -> Compare To Constant4/1
  Compare To Constant4/1 -> Logical Operator/3
  Memory1/1 -> Product4/2  "de-latch"
  [LKA_On] -> Memory2/1
  Memory2/1 -> Compare To Constant1/1
  Integrator/1 -> Compare To Constant/1
  Product6/1 -> Integrator/1, Integrator/2
  Compare To Constant1/1 -> Logical Operator/2
  Logical Operator/1 -> Data Type Conversion3/1  "first_and"
  Compare To Constant/1 -> Switch/1, Switch/2  "request_time"
  Data Type Conversion2/1 -> Product6/2, ADAS.Outputs.AP.AP_Ready/1, [AP_Ready]
  Data Type Conversion3/1 -> Integrator1/1, Integrator1/2, Compare To Constant5/1
  Compare To Constant5/1 -> Data Type Conversion2/1
  [Indicator_On] -> Compare To Constant6/1
  Compare To Constant6/1 -> Product4/3, Logical Operator/5
  Rate Transition/1 -> Demux3/1, Sum of Elements/1
  Sum of Elements/1 -> Gain3/1
  Gain3/1 -> Subtract4/2  "(a+b)/2"
  Demux3/2 -> Terminator/1
  Demux3/1 -> Subtract4/1
  Subtract4/1 -> Saturation/1  "error from center"
  [ADAS_Error] -> Compare To Zero/1
  Constant4/1 -> Product5/2
  Compare To Zero/1 -> Product5/1
  Product5/1 -> Logical Operator/6, Product4/5
  [Vicrt_Status] -> Compare To Constant8/1
  Compare To Constant8/1 -> Product4/4, Logical Operator/7
  [AP_Input_Driver_Steering] -> Rate Transition2/1
  Product/1 -> Discrete PID Controller2/1(In1)
  Rate Transition2/1 -> Discrete PID Controller2/3(In4)
  Discrete PID Controller2/1(Out1) -> Product1/2
  Rate Transition5/1 -> Product3/2, Subsystem/2(Input_Signal)
  [AP_Input_ACC_Ready] -> Logical Operator/1
  AP_Input_Driver_Throttle/1 -> Compare To Constant7/1
  Compare To Constant9/1 -> Product4/7, Terminator4/1
  [AP_Input_Driver_Brake] -> Compare To Constant9/1
  Compare To Constant7/1 -> Terminator3/1
  [ACC_Active] -> Product4/1
  Integrator1/1 -> Terminator1/1
  Mux/1 -> Rate Transition/1
  [AP_Input_laneGap_left] -> Mux/1
  [AP_Input_laneGap_right] -> Mux/2
  [AP_Error_fromcenter_derivate] -> Rate Transition8/1
  [AP_Input_Driver_Steering] -> Product2/1
  [AP_Input_Driver_Steering] -> Gain4/1
  [AP_Steer_Angle] -> Subtract2/1
  [AP_On] -> Rate Limiter1/1
  [AP_Error_fromcenter] -> Product/1
  Gain2/1 -> [AP_Steer_Angle]
  Memory/1 -> Product4/6
  Gain4/1 -> Subtract2/2
  Constant/1 -> [LDW_On], [LKA_On], [Indicator_On]
  [AP_Ready] -> Terminator2/1
  MATLAB Function/1(y) -> Reciprocal/1

== system auto_pilot_udp/AP/AP_Outputs ==
  Terminator : Terminator
  tag scope: AP_Output_Steer_Angle=global, AP_Output_Steer_Torque=global
  wires:
  [AP_Steer_Mode] -> [AP_Output_Steer_Torque]
  [AP_Steer_Angle] -> [AP_Output_Steer_Angle]
  [AP_Output_Steer_Torque] -> Terminator/1

== system auto_pilot_udp/INPUT/Inputs for CRT ==
  Clutch_manager : Subsystem
  Constant : Constant  Value=0
  Constant1 : Constant
  tag scope: brake_demand=global, clutch_demand=global, gear_demand=global, steering_angle_demand=global, steering_torque_demand=global, throttle_demand=global
  wires:
  [ACC_Output_Brake] -> [brake_demand]
  Constant/1 -> [steering_torque_demand]
  [AP_Output_Steer_Angle] -> [steering_angle_demand]
  Clutch_manager/1(clutch) -> [clutch_demand]
  [ACC_Output_Throttle] -> [throttle_demand]
  [ACC_Output_Throttle] -> Clutch_manager/1(throttle)
  Constant1/1 -> [gear_demand]

== system auto_pilot_udp/LDW/LDW_LaneGap_Warning1 ==
  In1 : Inport
  ADAS_Control_Mode : Constant  Value=ADAS_Control_Mode
  LDW_LaneGap_Warning : Constant  Value=LDW_LaneGap_Warning(1)
  LDW_LaneGap_Warning1 : Constant  Value=LDW_LaneGap_Warning(2)  VectorParams1D=off
  Multiport Switch : MultiPortSwitch  Inputs=2  DataPortForDefault=Additional data port  DiagnosticForDefault=None  SaturateOnIntegerOverflow=off  InputSameDT=off
  Relational Operator : RelationalOperator  Operator=<  OutDataTypeStr=boolean  InputSameDT=off
  Out1 : Outport  VectorParamsAs1DForOutWhenUnconnected=off
  wires:
  ADAS_Control_Mode/1 -> Multiport Switch/1
  Multiport Switch/1 -> Relational Operator/2
  Relational Operator/1 -> Out1/1
  In1/1 -> Relational Operator/1
  LDW_LaneGap_Warning/1 -> Multiport Switch/4, Multiport Switch/2
  LDW_LaneGap_Warning1/1 -> Multiport Switch/3

== system auto_pilot_udp/LKA/Discrete PID Controller ==
  In1 : Inport
  In2 : Inport  Port=2
  ADAS_Control_Mode : Constant  Value=ADAS_Control_Mode
  Demux : Demux  Outputs=3
  Discrete PID Controller : slpidlib/PID Controller  Controller=PID  Form=Parallel  TimeDomain=Discrete-time  UseExternalTs=off  SampleTime=1/LKA_Freq_Hz  IntegratorMethod=Forward Euler  FilterMethod=Forward Euler  ControllerParametersSource=external  P=LKA_P  I=LKA_I  UseKiTs=off  D=LKA_D  N=100  UseFilter=off  TunerSelectOption=Transfer Function Based (PID Tuner App)  InitialConditionSource=internal  InitialConditionForIntegrator=0  InitialConditionForFilter=0  DifferentiatorICPrevScaledInput=0  ExternalReset=either  TrackingMode=off  Kt=1  LimitOutput=off  SatLimitsSource=internal  UpperSaturationLimit=inf  LowerSaturationLimit=-inf  LinearizeAsGain=off  AntiWindupMode=clamping  Kb=1  LimitIntegrator=off  UpperIntegratorSaturationLimit=inf  LowerIntegratorSaturationLimit=-inf  POutMin=[]  POutMax=[]  IOutMin=[]  IOutMax=[]  DOutMin=[]  DOutMax=[]  NOutMin=[]  NOutMax=[]  SumOutMin=[]  SumOutMax=[]  SaturationOutMin=[]  SaturationOutMax=[]  PParamMin=[]  PParamMax=[]  IParamMin=[]  IParamMax=[]  DParamMin=[]  DParamMax=[]  NParamMin=[]  NParamMax=[]  KbParamMin=[]  KbParamMax=[]  KtParamMin=[]  KtParamMax=[]  KbOutMin=[]  KbOutMax=[]  KtOutMin=[]  KtOutMax=[]  IntegratorOutMin=[]  IntegratorOutMax=[]  FilterOutMin=[]  FilterOutMax=[]  SumI1OutMin=[]  SumI1OutMax=[]  SumI2OutMin=[]  SumI2OutMax=[]  SumI3OutMin=[]  SumI3OutMax=[]  SumI4OutMin=[]  SumI4OutMax=[]  SumDOutMin=[]  SumDOutMax=[]  DifferentiatorOutMin=[]  DifferentiatorOutMax=[]  FilterDiffOutCoefMin=[]  FilterDiffOutCoefMax=[]  ReciprocalOutMin=[]  ReciprocalOutMax=[]  SumDenOutMin=[]  SumDenOutMax=[]  SumNumOutMin=[]  SumNumOutMax=[]  DivideOutMin=[]  DivideOutMax=[]  UdiffTsProdOutMin=[]  UdiffTsProdOutMax=[]  NTsProdOutMin=[]  NTsProdOutMax=[]  UintegralTsProdOutMin=[]  UintegralTsProdOutMax=[]  UngainTsProdOutMin=[]  UngainTsProdOutMax=[]  ClampingZeroOutDataTypeStr=Inherit: Inherit via back propagation  ClampingZeroOutMin=[]  ClampingZeroOutMax=[]  FilterDenConstantOutDataTypeStr=Inherit: Inherit via back propagation  FilterDenConstantOutMin=[]  FilterDenConstantOutMax=[]  PCopyOutDataTypeStr=Inherit: Inherit via back propagation  PCopyOutMin=[]  PCopyOutMax=[]  NCopyOutDataTypeStr=Inherit: Inherit via back propagation  NCopyOutMin=[]  NCopyOutMax=[]  IntegratorContinuousStateAttributes=''  IntegratorStateMustResolveToSignalObject=off  IntegratorRTWStateStorageClass=Auto  FilterContinuousStateAttributes=''  FilterStateMustResolveToSignalObject=off  FilterRTWStateStorageClass=Auto  ParallelPVariant=ExternalParameters  IdealPVariant=Disabled  IVariant=ExternalParameters  DVariant=ExternalParameters  IntegratorVariant=Discrete  SatVariant=Disabled  AWVariant=Passthrough  PCopyVariant=Disabled  TRVariant=Disabled  FdbkBlocksVariant=Forward  IdealPFdbkVariant=Disabled  SatFdbkVariant=Disabled  DerivativeFilterVariant=Differentiator  NVariant=Passthrough  NCopyVariant=Disabled_SignalSpec  FilterICVariant=InternalICsDifferentiator  IntegratorICVariant=InternalICs  ExternalResetVariant=ExternalReset  TRSumVariant=Passthrough  SumFdbkVariant=Disabled  SumVariant=Sum_PID  TsampFilterVariant=InternalTs  TsampNgainVariant=Passthrough  TsampIntegralVariant=Passthrough  ExternalSaturationOutDataTypeStr=Inherit: Same as second input
  LKA_D(1) : Constant  Value=LKA_D(1)
  LKA_D(1)1 : Constant  Value=LKA_D(2)
  LKA_I(1) : Constant  Value=LKA_I(1)
  LKA_I(1)1 : Constant  Value=LKA_I(2)
  LKA_P(1) : Constant  Value=LKA_P(1)
  LKA_P(1)1 : Constant  Value=LKA_P(2)
  Multiport Switch : MultiPortSwitch  Inputs=2  DataPortForDefault=Additional data port  DiagnosticForDefault=None  SaturateOnIntegerOverflow=off  InputSameDT=off
  Mux : Mux  Inputs=3
  Mux1 : Mux  Inputs=3
  Out1 : Outport  VectorParamsAs1DForOutWhenUnconnected=off
  wires:
  In1/1 -> Discrete PID Controller/1
  In2/1 -> Discrete PID Controller/5
  Discrete PID Controller/1 -> Out1/1
  LKA_P(1)/1 -> Mux/1
  ADAS_Control_Mode/1 -> Multiport Switch/1
  Demux/2 -> Discrete PID Controller/3
  Demux/3 -> Discrete PID Controller/4
  Demux/1 -> Discrete PID Controller/2
  Mux1/1 -> Multiport Switch/3
  Mux/1 -> Multiport Switch/4, Multiport Switch/2
  LKA_I(1)/1 -> Mux/2
  LKA_D(1)/1 -> Mux/3
  LKA_P(1)1/1 -> Mux1/1
  LKA_I(1)1/1 -> Mux1/2
  LKA_D(1)1/1 -> Mux1/3
  Multiport Switch/1 -> Demux/1

== system auto_pilot_udp/LKA/LKA_Lane_Gap_Activate ==
  In1 : Inport
  ADAS_Control_Mode : Constant  Value=ADAS_Control_Mode
  LKA_Lane_Gap_Activate : Constant  Value=LKA_Lane_Gap_Activate(1)
  LKA_Lane_Gap_Activate2 : Constant  Value=LKA_Lane_Gap_Activate(2)  VectorParams1D=off
  Multiport Switch : MultiPortSwitch  Inputs=2  DataPortForDefault=Additional data port  DiagnosticForDefault=None  SaturateOnIntegerOverflow=off  InputSameDT=off
  Relational Operator : RelationalOperator  Operator=<  OutDataTypeStr=boolean  InputSameDT=off
  Out1 : Outport  VectorParamsAs1DForOutWhenUnconnected=off
  wires:
  ADAS_Control_Mode/1 -> Multiport Switch/1
  Multiport Switch/1 -> Relational Operator/2
  Relational Operator/1 -> Out1/1
  In1/1 -> Relational Operator/1
  LKA_Lane_Gap_Activate/1 -> Multiport Switch/4, Multiport Switch/2
  LKA_Lane_Gap_Activate2/1 -> Multiport Switch/3

== system auto_pilot_udp/LKA/Subsystem ==
  Clock : Inport
  Input_Signal : Inport  Port=2
  Delay : Delay  DelayLength=1000/LKA_Freq_Hz  InitialCondition=-1/LKA_Freq_Hz
  Delay1 : Delay  DelayLength=1000/LKA_Freq_Hz
  Delay2 : Delay  DelayLength=1000/LKA_Freq_Hz
  Lookup Table Dynamic : simulink/Lookup Tables/Lookup Table Dynamic  LookUpMeth=Interpolation-Use End Values  OutDataType=fixdt('double')  OutScaling=[]  OutputDataTypeScalingMode=Specify via dialog  OutDataTypeStr=fixdt('double')  DoSatur=off
  Vector Concatenate : Concatenate
  Vector Concatenate1 : Concatenate
  Zero-Order Hold1 : ZeroOrderHold  SampleTime=1/LKA_Freq_Hz
  Zero-Order Hold2 : ZeroOrderHold  SampleTime=1/LKA_Freq_Hz
  Zero-Order Hold3 : ZeroOrderHold  SampleTime=1e-3
  Zero-Order Hold4 : ZeroOrderHold  SampleTime=1e-3
  1kHz_Interpolation : Outport  VectorParamsAs1DForOutWhenUnconnected=off
  wires:
  Input_Signal/1 -> Zero-Order Hold1/1
  Zero-Order Hold1/1 -> Zero-Order Hold4/1
  Zero-Order Hold3/1 -> Delay/1, Vector Concatenate/2
  Zero-Order Hold2/1 -> Zero-Order Hold3/1
  Delay/1 -> Vector Concatenate/1
  Delay1/1 -> Lookup Table Dynamic/1
  Delay2/1 -> Vector Concatenate1/1
  Zero-Order Hold4/1 -> Delay2/1, Vector Concatenate1/2
  Vector Concatenate1/1 -> Lookup Table Dynamic/3
  Vector Concatenate/1 -> Lookup Table Dynamic/2
  Clock/1 -> Delay1/1, Zero-Order Hold2/1
  Lookup Table Dynamic/1 -> 1kHz_Interpolation/1

== system auto_pilot_udp/OUTPUT/VI-CarRealTime_Outputs ==
  Gain : Gain  Gain=1/2
  Log_bus : BusSelector  OutputSignals=VI_CarRealTime:Outputs:chassis_velocities:longitudinal,VI_CarRealTime:Outputs:driver_demands:steering,VI_CarRealTime:Outputs:Wheel:Spindle_Steer:L1,VI_CarRealTime:Outputs:Wheel:Spindle_Steer:R1,VI_CarRealTime:Outputs:driver_demands:throttle,VI_CarRealTime:Outputs:driver_demands:brake,VI_CarRealTime:Outputs:chassis_accelerations:longitudinal,VI_CarRealTime:Outputs:chassis_accelerations:lateral,VI_CarRealTime:Outputs:Steering_System:DriveSim_Steering_Feedback_Torque  OutputAsBus=on
  Scope : Scope  NumInputPorts=2
  Sum : Sum
  Terminator : Terminator
  internal_bus : BusSelector  OutputSignals=VI_CarRealTime:Outputs:chassis_velocities:longitudinal,VI_CarRealTime:Outputs:driver_demands:steering,VI_CarRealTime:Outputs:Wheel:Spindle_Steer:L1,VI_CarRealTime:Outputs:Wheel:Spindle_Steer:R1,VI_CarRealTime:Outputs:driver_demands:throttle,VI_CarRealTime:Outputs:driver_demands:brake,VI_CarRealTime:Outputs:chassis_accelerations:longitudinal,VI_CarRealTime:Outputs:chassis_accelerations:lateral,VI_CarRealTime:Outputs:Steering_System:DriveSim_Steering_Feedback_Torque
  tag scope: Driver_Brake=global, Driver_Steering=global, Driver_Throttle=global, Front_Axle_Steer=global, Lateral_Accelerations=global, Longitudinal_Accelerations=global, Steering_feedback_torque=global, Vehicle_Speed=global
  wires:
  internal_bus/9 -> [Steering_feedback_torque]  "<VI_CarRealTime:Outputs:Steering_System:DriveSim_Steering_Feedback_Torque>"
  internal_bus/8 -> [Lateral_Accelerations]  "<VI_CarRealTime:Outputs:chassis_accelerations:lateral>"
  internal_bus/7 -> [Longitudinal_Accelerations]  "<VI_CarRealTime:Outputs:chassis_accelerations:longitudinal>"
  internal_bus/6 -> [Driver_Brake]  "<VI_CarRealTime:Outputs:driver_demands:brake>"
  internal_bus/5 -> [Driver_Throttle]  "<VI_CarRealTime:Outputs:driver_demands:throttle>"
  Gain/1 -> [Front_Axle_Steer]
  Sum/1 -> Gain/1
  internal_bus/4 -> Sum/2  "<VI_CarRealTime:Outputs:Wheel:Spindle_Steer:R1>"
  internal_bus/3 -> Sum/1  "<VI_CarRealTime:Outputs:Wheel:Spindle_Steer:L1>"
  [Vehicle_outputs] -> internal_bus/1, Log_bus/1
  internal_bus/2 -> [Driver_Steering], Scope/2  "<VI_CarRealTime:Outputs:driver_demands:steering>"
  Log_bus/1 -> Terminator/1  "VI_CarRealTime_selection"
  internal_bus/1 -> [Vehicle_Speed], Scope/1  "<VI_CarRealTime:Outputs:chassis_velocities:longitudinal>"
